simulink subsystem "Controller"  (R2022b)
settings: Solver=VariableStepAuto  StartTime=0.0  StopTime=10.0  RelTol=1e-3
settings Model: Creator=Sahil Gaurkar  LastModifiedBy=Sahil Gaurkar

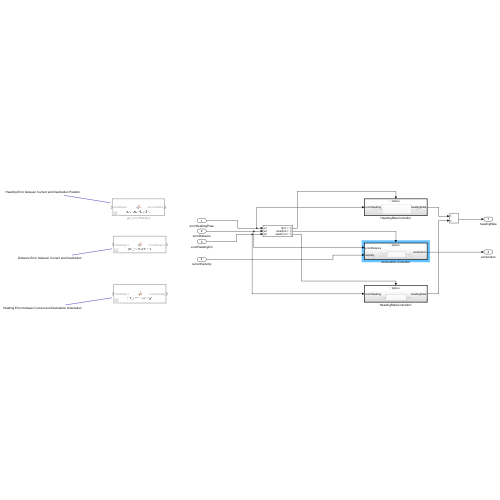
[thumbnail: Simulink's stored preview of the top-level diagram]
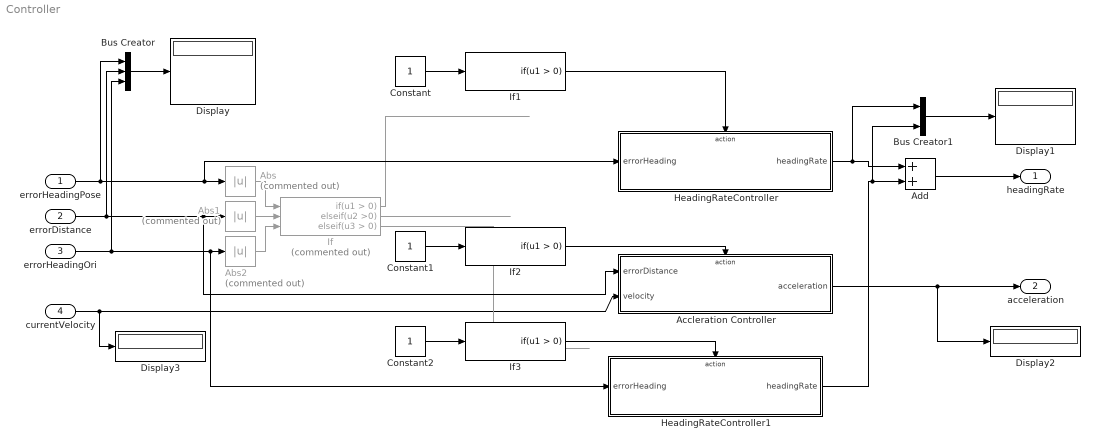
== system Controller ==
  errorHeadingPose : Inport
  errorDistance : Inport  Port=2
  errorHeadingOri : Inport  Port=3
  currentVelocity : Inport  Port=4
  Abs : Abs  Commented=on  SaturateOnIntegerOverflow=off
  Abs1 : Abs  Commented=on  SaturateOnIntegerOverflow=off
  Abs2 : Abs  Commented=on  SaturateOnIntegerOverflow=off
  Accleration Controller : Subsystem  TreatAsAtomicUnit=on
  Add : Sum
  Bus Creator : BusCreator  Inputs=3
  Bus Creator1 : BusCreator  Inputs=2
  Constant : Constant
  Constant1 : Constant
  Constant2 : Constant
  Display{,1..3} (4 alike) : Display
  HeadingRateController : Subsystem  TreatAsAtomicUnit=on
  HeadingRateController1 : Subsystem  TreatAsAtomicUnit=on
  If : If  Commented=on  NumInputs=3  ElseIfExpressions=u2 >0, u3 > 0  ShowElse=off
  If1 : If  ShowElse=off
  If2 : If  ShowElse=off
  If3 : If  ShowElse=off
  headingRate : Outport
  acceleration : Outport  Port=2
  wires:
  Bus Creator1/1 -> Display1/1
  Bus Creator/1 -> Display/1
  Abs2/1 -> If/3
  Abs1/1 -> If/2
  Abs/1 -> If/1
  currentVelocity/1 -> Accleration Controller/2(velocity), Display3/1
  HeadingRateController/1(headingRate) -> Bus Creator1/1, Add/1
  errorHeadingOri/1 -> Bus Creator/3, Abs2/1, HeadingRateController1/1(errorHeading)
  If/1 -> ?
  Add/1 -> headingRate/1
  If/2 -> ?
  HeadingRateController1/1(headingRate) -> Bus Creator1/2, Add/2
  If/3 -> ?
  Accleration Controller/1(acceleration) -> acceleration/1, Display2/1
  errorHeadingPose/1 -> Bus Creator/1, Abs/1, HeadingRateController/1(errorHeading)
  errorDistance/1 -> Bus Creator/2, Accleration Controller/1(errorDistance), Abs1/1
  Constant/1 -> If1/1
  Constant1/1 -> If2/1
  Constant2/1 -> If3/1
  If1/1 -> HeadingRateController/Action
  If2/1 -> Accleration Controller/Action
  If3/1 -> HeadingRateController1/Action

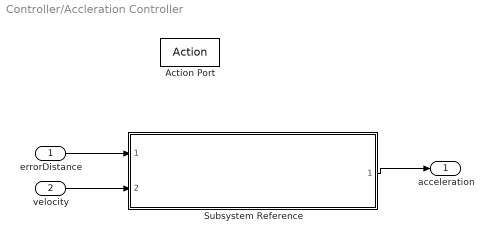
== system Controller/Accleration Controller ==
  errorDistance : Inport
  velocity : Inport  Port=2
  Action Port : ActionPort
  Subsystem Reference : Subsystem  ReferencedSubsystem=AcclerationController
  acceleration : Outport
  wires:
  velocity/1 -> Subsystem Reference/2
  Subsystem Reference/1 -> acceleration/1
  errorDistance/1 -> Subsystem Reference/1

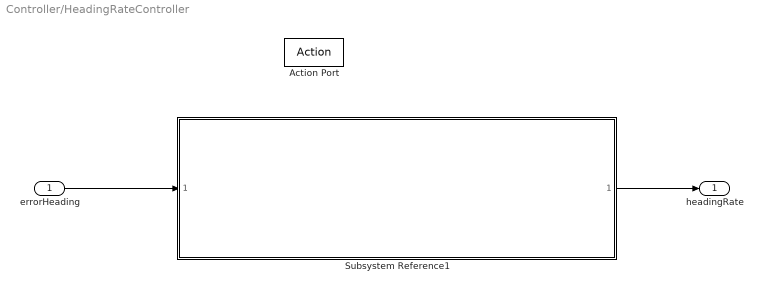
== system Controller/HeadingRateController ==
  errorHeading : Inport
  Action Port : ActionPort
  Subsystem Reference1 : Subsystem  ReferencedSubsystem=HeadingRateController
  headingRate : Outport
  wires:
  Subsystem Reference1/1 -> headingRate/1
  errorHeading/1 -> Subsystem Reference1/1

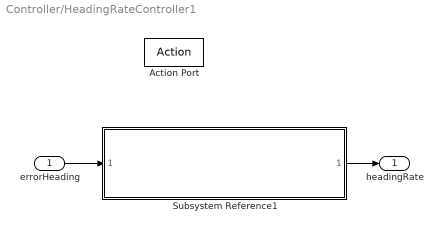
== system Controller/HeadingRateController1 ==
  errorHeading : Inport
  Action Port : ActionPort
  Subsystem Reference1 : Subsystem  ReferencedSubsystem=HeadingRateController
  headingRate : Outport
  wires:
  Subsystem Reference1/1 -> headingRate/1
  errorHeading/1 -> Subsystem Reference1/1
